simulink model "test2_model"  (R2024b)
settings: Solver=ode1  StartTime=0.0  StopTime=25  FixedStep=0.001  RelTol=1e-3
values from neighbouring files (symbols this model uses):
  t_freq = [0.1, 100]    [test_2.m]
  theta0 = 0    [Project1_Part1_Code_revision_current.m]    (also in test_2.m)
  torque_mode = [0,1]    [Project1_Part1_Code_revision_current.m]    (also in test_2.m)
undefined symbols (not defined in the file or in its folder): b, J, omega0, tau0
settings Model: Creator=jacobcody  LastModifiedBy=mjsch

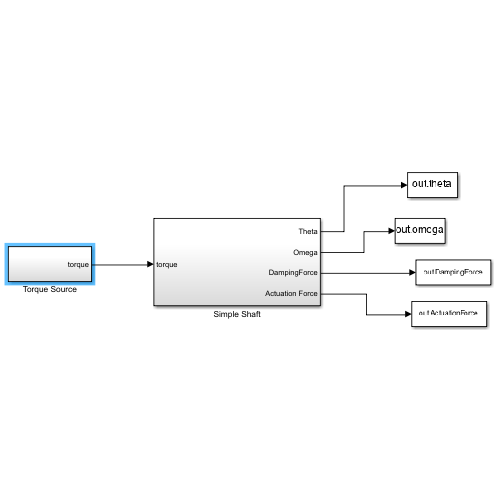
[thumbnail: Simulink's stored preview of the top-level diagram]
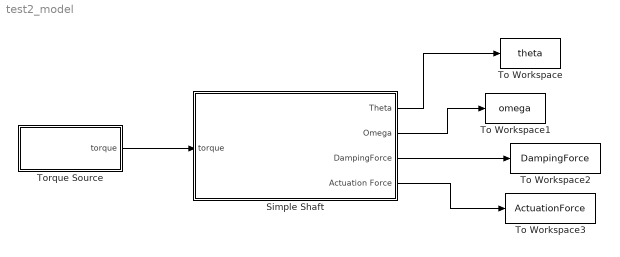
== system test2_model ==
  Simple Shaft : Subsystem
  To Workspace : ToWorkspace  VariableName=theta  SaveFormat=Timeseries  SampleTime=-1
  To Workspace1 : ToWorkspace  VariableName=omega  SaveFormat=Timeseries  SampleTime=-1
  To Workspace2 : ToWorkspace  VariableName=DampingForce  SaveFormat=Timeseries  SampleTime=-1
  To Workspace3 : ToWorkspace  VariableName=ActuationForce  SaveFormat=Timeseries  SampleTime=-1
  Torque Source : Subsystem
  wires:
  Torque Source/1(torque) -> Simple Shaft/1(torque)
  Simple Shaft/1(Theta) -> To Workspace/1
  Simple Shaft/2(Omega) -> To Workspace1/1
  Simple Shaft/3(DampingForce) -> To Workspace2/1
  Simple Shaft/4(Actuation Force) -> To Workspace3/1

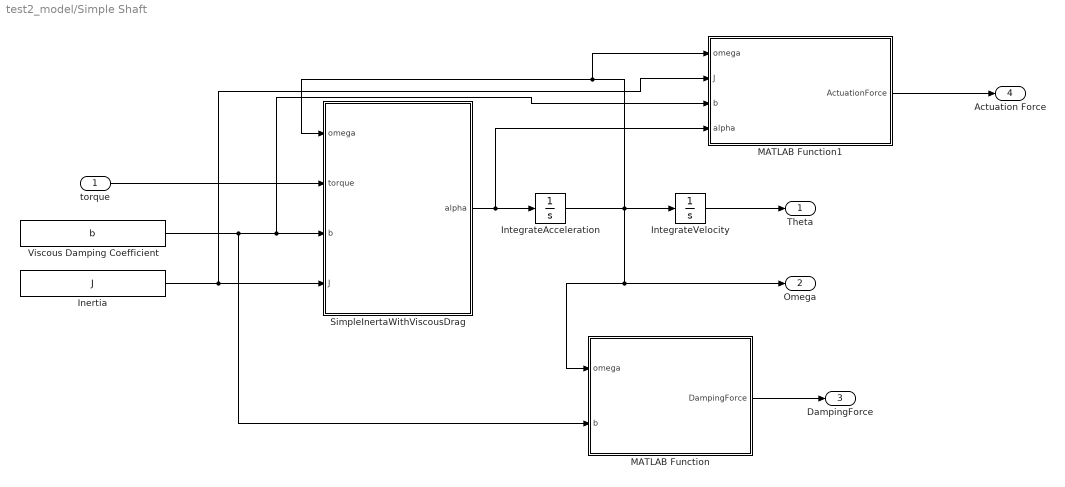
== system test2_model/Simple Shaft ==
  torque : Inport
  Inertia : Constant  Value=J
  IntegrateAcceleration : Integrator  InitialCondition=omega0
  IntegrateVelocity : Integrator  InitialCondition=theta0
  MATLAB Function : MATLAB Function  TreatAsAtomicUnit=on
  MATLAB Function1 : MATLAB Function  TreatAsAtomicUnit=on
  SimpleInertaWithViscousDrag : MATLAB Function  TreatAsAtomicUnit=on
  Viscous Damping Coefficient : Constant  Value=b
  Theta : Outport
  Omega : Outport  Port=2
  DampingForce : Outport  Port=3
  Actuation Force : Outport  Port=4
  wires:
  IntegrateAcceleration/1 -> MATLAB Function1/1(omega), SimpleInertaWithViscousDrag/1(omega), Omega/1, MATLAB Function/1(omega), IntegrateVelocity/1
  IntegrateVelocity/1 -> Theta/1
  SimpleInertaWithViscousDrag/1(alpha) -> MATLAB Function1/4(alpha), IntegrateAcceleration/1
  torque/1 -> SimpleInertaWithViscousDrag/2(torque)
  Viscous Damping Coefficient/1 -> MATLAB Function/2(b), MATLAB Function1/3(b), SimpleInertaWithViscousDrag/3(b)
  Inertia/1 -> MATLAB Function1/2(J), SimpleInertaWithViscousDrag/4(J)
  MATLAB Function/1(DampingForce) -> DampingForce/1
  MATLAB Function1/1(ActuationForce) -> Actuation Force/1

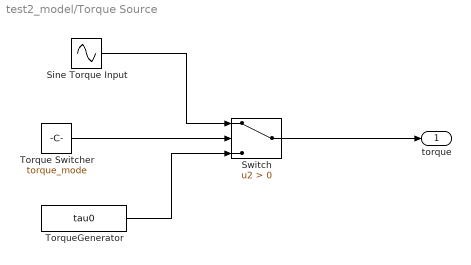
== system test2_model/Torque Source ==
  Sine Torque Input : Sin  Frequency=t_freq  SampleTime=0
  Switch : Switch  Criteria=u2 > Threshold  SaturateOnIntegerOverflow=off  InputSameDT=off
  Torque Switcher : Constant  Value=torque_mode
  TorqueGenerator : Constant  Value=tau0
  torque : Outport
  wires:
  Switch/1 -> torque/1
  Sine Torque Input/1 -> Switch/1
  TorqueGenerator/1 -> Switch/3
  Torque Switcher/1 -> Switch/2

== matlab function test2_model/Simple Shaft/MATLAB Function ==
  data: omega input; DampingForce output; b input
function DampingForce = fcn(omega,b)
DampingForce = omega * b;

== matlab function test2_model/Simple Shaft/SimpleInertaWithViscousDrag ==
  data: omega input; torque input; alpha output; b input; J input
function alpha = fcn(omega, torque,b, J)
alpha = (torque - omega * b)/J;

== matlab function test2_model/Simple Shaft/MATLAB Function1 ==
  data: omega input; ActuationForce output; J input; b input; alpha input
function ActuationForce = fcn(omega, J, b, alpha)

ActuationForce = J * alpha + b * omega;
